simulink model "Simulation_Kinematic_LevMar_InsDiMov"  (R2022a)
settings: Solver=VariableStepAuto  StartTime=0.0  StopTime=0.5  MaxStep=0.01  RelTol=1e-3
values from neighbouring files (symbols this model uses):
  K = 20 * eye(6)    [Kinematic.m]
  mu0 = 1/1000    (= 0.001)    [Kinematic.m]
libraries: robotcorelib x2, robotmaniplib x1
settings Model: Creator=ramti  LastModifiedBy=v
settings SolverCC: AlgebraicLoopSolver=TrustRegion
settings DebuggingCC: UnconnectedInputMsg=warning  UnconnectedOutputMsg=warning  UnconnectedLineMsg=warning  SFMachineParentedDataDiag=warning
settings RTWCC: DLArmComputeVersion=19.05

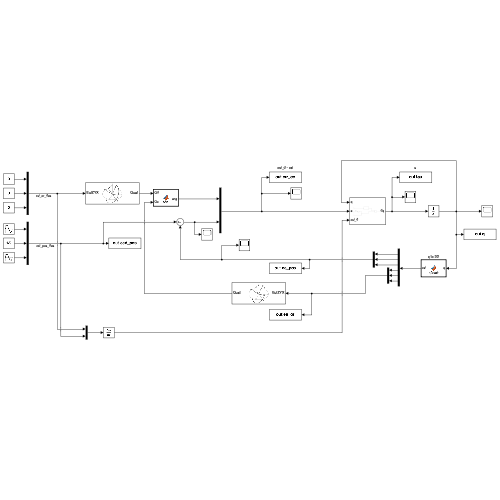
[thumbnail: Simulink's stored preview of the top-level diagram]
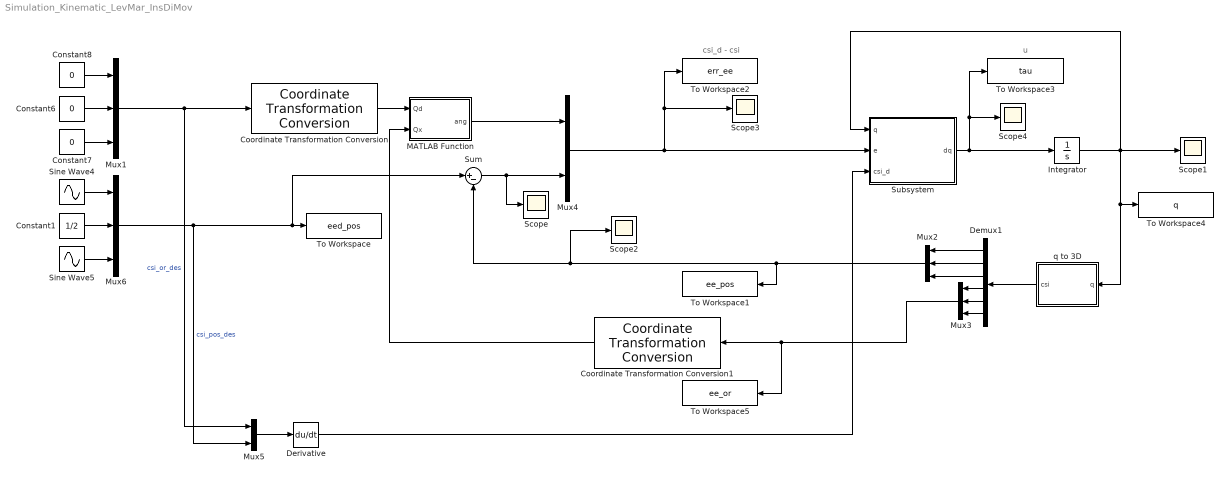
== system Simulation_Kinematic_LevMar_InsDiMov ==
  note: csi_d - csi
  note: u
  Constant1 : Constant  Value=1/2
  Constant6 : Constant  Value=0
  Constant7 : Constant  Value=0
  Constant8 : Constant  Value=0
  Coordinate Transformation Conversion : robotcorelib/Coordinate Transformation Conversion  InputRepresentation=Euler Angles  InputEulerSequence=ZYX  ShowTrVecInputPort=on  OutputRepresentation=Quaternion  OutputEulerSequence=ZYX  ShowTrVecOutputPort=on  SimulateUsing=Interpreted execution
      settings: SourceProductBaseCode=RO,NV,RR,UV
  Coordinate Transformation Conversion1 : robotcorelib/Coordinate Transformation Conversion  InputRepresentation=Euler Angles  InputEulerSequence=ZYX  ShowTrVecInputPort=on  OutputRepresentation=Quaternion  OutputEulerSequence=ZYX  ShowTrVecOutputPort=on  SimulateUsing=Interpreted execution
      settings: SourceProductBaseCode=RO,NV,RR,UV
  Demux1 : Demux  Outputs=6
  Derivative : Derivative
  Integrator : Integrator  InitialCondition=zeros(6,1)
  MATLAB Function : MATLAB Function  TreatAsAtomicUnit=on
  Mux{1..3,6} (4 alike) : Mux  Inputs=3
  Mux4 : Mux  Inputs=2
  Mux5 : Mux  Inputs=2
  Scope{,1..4} (5 alike) : Scope
  Sine Wave4 : Sin  Amplitude=1/2  Frequency=pi/3  SampleTime=0
  Sine Wave5 : Sin  Amplitude=1/2  Frequency=pi/3  Phase=pi/2  SampleTime=0
  Subsystem : Subsystem
      settings: OpenFcn="mdl_puma560_simpl;    % Modello Peter Corke semplificato"
  Sum : Sum  Inputs=|+-
  To Workspace : ToWorkspace  VariableName=eed_pos  SaveFormat=Timeseries  SampleTime=-1
  To Workspace1 : ToWorkspace  VariableName=ee_pos  SaveFormat=Structure With Time  SampleTime=-1
  To Workspace2 : ToWorkspace  VariableName=err_ee  SaveFormat=Structure With Time  SampleTime=-1
  To Workspace3 : ToWorkspace  VariableName=tau  SaveFormat=Structure With Time  SampleTime=-1
  To Workspace4 : ToWorkspace  VariableName=q  SaveFormat=Structure With Time  SampleTime=-1
  To Workspace5 : ToWorkspace  VariableName=ee_or  SaveFormat=Structure With Time  SampleTime=-1
  q to 3D : MATLAB Function  TreatAsAtomicUnit=on
  wires:
  Sum/1 -> Scope/1, Mux4/2
  Demux1/1 -> Mux2/1
  Mux4/1 -> Scope3/1, To Workspace2/1, Subsystem/2(e)
  Demux1/6 -> Mux3/3
  Demux1/5 -> Mux3/2
  MATLAB Function/1(ang) -> Mux4/1
  Demux1/2 -> Mux2/2
  Integrator/1 -> Scope1/1, To Workspace4/1, q to 3D/1(q), Subsystem/1(q)
  Demux1/4 -> Mux3/1
  Demux1/3 -> Mux2/3
  q to 3D/1(csi) -> Demux1/1
  Coordinate Transformation Conversion1/1 -> MATLAB Function/2(Qx)
  Coordinate Transformation Conversion/1 -> MATLAB Function/1(Qd)
  Derivative/1 -> Subsystem/3(csi_d)
  Mux5/1 -> Derivative/1
  Mux6/1 -> Mux5/2, To Workspace/1, Sum/1  "csi_pos_des"
  Subsystem/1(dq) -> Scope4/1, To Workspace3/1, Integrator/1
  Mux2/1 -> To Workspace1/1, Scope2/1, Sum/2
  Mux3/1 -> To Workspace5/1, Coordinate Transformation Conversion1/1
  Sine Wave5/1 -> Mux6/3
  Sine Wave4/1 -> Mux6/1
  Constant1/1 -> Mux6/2
  Constant7/1 -> Mux1/3
  Constant6/1 -> Mux1/2
  Constant8/1 -> Mux1/1
  Mux1/1 -> Mux5/1, Coordinate Transformation Conversion/1  "csi_or_des"

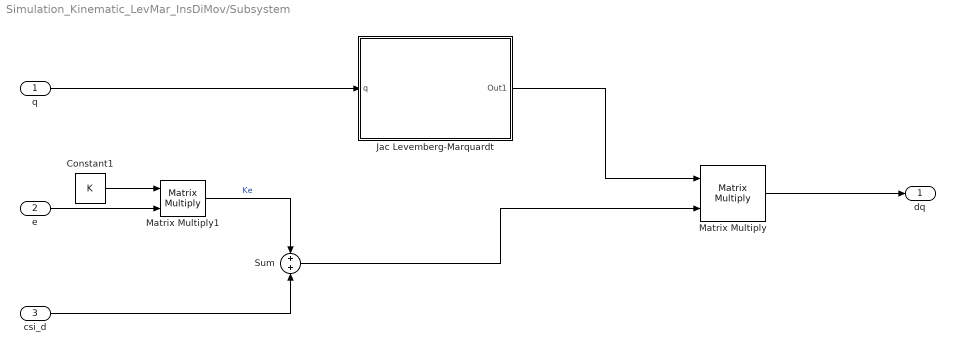
== system Simulation_Kinematic_LevMar_InsDiMov/Subsystem ==
  q : Inport
  e : Inport  Port=2
  csi_d : Inport  Port=3
  Constant1 : Constant  Value=K  VectorParams1D=off
  Jac Levemberg-Marquardt : Subsystem
  Matrix Multiply : Product  Inputs=**  Multiplication=Matrix(*)
  Matrix Multiply1 : Product  Multiplication=Matrix(*)
  Sum : Sum
  dq : Outport
  wires:
  Jac Levemberg-Marquardt/1(Out1) -> Matrix Multiply/1
  Matrix Multiply/1 -> dq/1
  q/1 -> Jac Levemberg-Marquardt/1(q)
  Matrix Multiply1/1 -> Sum/1  "Ke"
  csi_d/1 -> Sum/2
  Sum/1 -> Matrix Multiply/2
  e/1 -> Matrix Multiply1/2
  Constant1/1 -> Matrix Multiply1/1

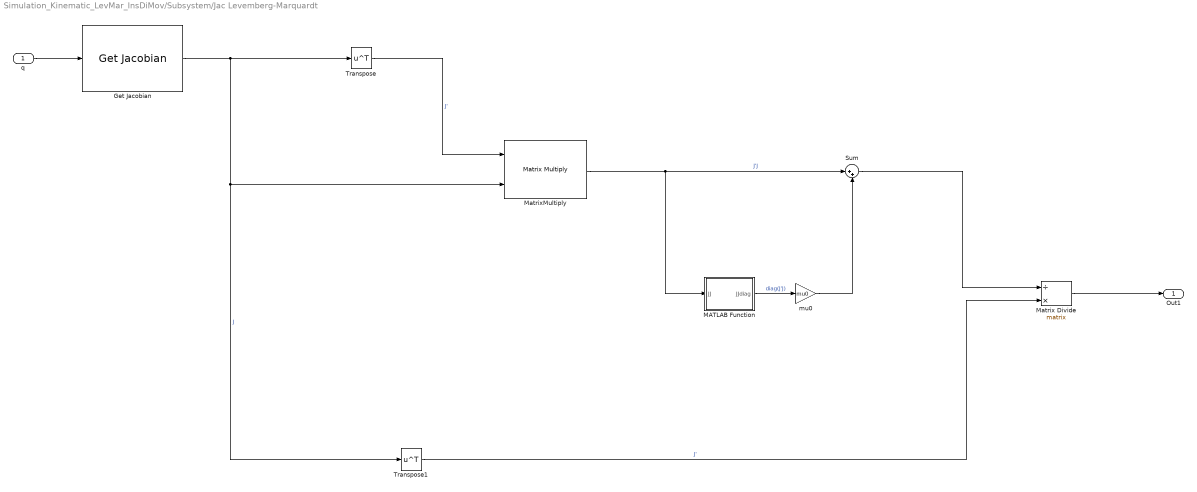
== system Simulation_Kinematic_LevMar_InsDiMov/Subsystem/Jac Levemberg-Marquardt ==
  q : Inport
  Get Jacobian : robotmaniplib/Get Jacobian  RigidBodyTree=robot_p560  EndEffector=body6  SimulateUsing=Interpreted execution
      settings: SourceProductBaseCode=RO
  MATLAB Function : MATLAB Function  TreatAsAtomicUnit=on
  Matrix Divide : Product  Inputs=/*  Multiplication=Matrix(*)
  MatrixMultiply : Product  Multiplication=Matrix(*)
  Sum : Sum  Inputs=|++
  Transpose : Math  Operator=transpose
  Transpose1 : Math  Operator=transpose
  mu0 : Gain  Gain=mu0
  Out1 : Outport
  wires:
  Transpose/1 -> MatrixMultiply/1  "J'"
  MatrixMultiply/1 -> MATLAB Function/1(JJ), Sum/1  "J'J"
  Sum/1 -> Matrix Divide/1
  Get Jacobian/1 -> Transpose1/1, MatrixMultiply/2, Transpose/1  "J"
  Transpose1/1 -> Matrix Divide/2  "J'"
  Matrix Divide/1 -> Out1/1
  MATLAB Function/1(JJdiag) -> mu0/1  "diag(J'J)"
  mu0/1 -> Sum/2
  q/1 -> Get Jacobian/1

== matlab function Simulation_Kinematic_LevMar_InsDiMov/q to 3D ==
  data: q input; csi output
function csi = q2cart(q)

% coder.extrinsic('eval','rotm2eul');

csi = zeros(6,1);

q1 = q(1); q2 = q(2); q3 = q(3); q4 = q(4); q5 = q(5); q6 = q(6); 

% dh = [0 0 0 q1; 0 -pi/2 0 q2; 0.432 0 0.149 q3; 0.0203 -pi/2 0 q4; 0 pi/2 0.433 q5; 0 -pi/2 0 q6];
% Denavit-Hartenberg
a2 = 0.4318;    a3 = 0.0203;
d3 = 0.15005;   d4 = 0.4318;
    
dh = [0     pi/2        0       q1;
      a2    0           0       q2;
      a3    -pi/2       d3      q3;
      0     pi/2        d4      q4;
      0     -pi/2       0       q5;
      0     0           0       q6];
  
A00 = eye(4);

A1 = [cos(dh(1,4)), -sin(dh(1,4))*cos(dh(1,2)), sin(dh( 1,4))*sin(dh( 1,2)),  dh( 1,1)*cos(dh( 1,4)); sin(dh( 1,4)), cos(dh( 1,4))*cos(dh( 1,2)), -cos(dh( 1,4))*sin(dh( 1,2)), dh( 1,1)*sin(dh( 1,4));0, sin(dh( 1,2)), cos(dh( 1,2)), dh(1,3);0, 0, 0, 1];
A2 = [cos(dh(2,4)), -sin(dh(2,4))*cos(dh(2,2)), sin(dh( 2,4))*sin(dh( 2,2)),  dh( 2,1)*cos(dh( 2,4)); sin(dh( 2,4)), cos(dh( 2,4))*cos(dh( 2,2)), -cos(dh( 2,4))*sin(dh( 2,2)), dh( 2,1)*sin(dh( 2,4));0, sin(dh( 2,2)), cos(dh( 2,2)), dh(2,3);0, 0, 0, 1];
A3 = [cos(dh(3,4)), -sin(dh(3,4))*cos(dh(3,2)), sin(dh( 3,4))*sin(dh( 3,2)),  dh( 3,1)*cos(dh( 3,4)); sin(dh( 3,4)), cos(dh( 3,4))*cos(dh( 3,2)), -cos(dh( 3,4))*sin(dh( 3,2)), dh( 3,1)*sin(dh( 3,4));0, sin(dh( 3,2)), cos(dh( 3,2)), dh(3,3);0, 0, 0, 1];
A4 = [cos(dh(4,4)), -sin(dh(4,4))*cos(dh(4,2)), sin(dh( 4,4))*sin(dh( 4,2)),  dh( 4,1)*cos(dh( 4,4)); sin(dh( 4,4)), cos(dh( 4,4))*cos(dh( 4,2)), -cos(dh( 4,4))*sin(dh( 4,2)), dh( 4,1)*sin(dh( 4,4));0, sin(dh( 4,2)), cos(dh( 4,2)), dh(4,3);0, 0, 0, 1];
A5 = [cos(dh(5,4)), -sin(dh(5,4))*cos(dh(5,2)), sin(dh( 5,4))*sin(dh( 5,2)),  dh( 5,1)*cos(dh( 5,4)); sin(dh( 5,4)), cos(dh( 5,4))*cos(dh( 5,2)), -cos(dh( 5,4))*sin(dh( 5,2)), dh( 5,1)*sin(dh( 5,4));0, sin(dh( 5,2)), cos(dh( 5,2)), dh(5,3);0, 0, 0, 1];
A6 = [cos(dh(6,4)), -sin(dh(6,4))*cos(dh(6,2)), sin(dh( 6,4))*sin(dh( 6,2)),  dh( 6,1)*cos(dh( 6,4)); sin(dh( 6,4)), cos(dh( 6,4))*cos(dh( 6,2)), -cos(dh( 6,4))*sin(dh( 6,2)), dh( 6,1)*sin(dh( 6,4));0, sin(dh( 6,2)), cos(dh( 6,2)), dh(6,3);0, 0, 0, 1];

A06 = A00*A1*A2*A3*A4*A5*A6;

% for (i=1:6)
%    
%     eval(sprintf('A%d= [cos(dh(%d,4)), -sin(dh(%d,4))*cos(dh(%d,2)), sin(dh( %d,4))*sin(dh( %d,2)),  dh( %d,1)*cos(dh( %d,4)); sin(dh( %d,4)), cos(dh( %d,4))*cos(dh( %d,2)), -cos(dh( %d,4))*sin(dh( %d,2)), dh( %d,1)*sin(dh( %d,4));0, sin(dh( %d,2)), cos(dh( %d,2)), dh(%d,3);0, 0, 0, 1];',i*ones(1,18)))
% 
%     eval(sprintf('A0%d = A0%d*A%d;',i,i-1,i))
% end

xi_hom = A06*[0;0;0;1];

R_xi = A06(1:3,1:3);
csi = [xi_hom(1:3);transpose(rotm2eul(R_xi))];

== matlab function Simulation_Kinematic_LevMar_InsDiMov/MATLAB Function ==
  data: Qd input; ang output; Qx input
function ang = fcn(Qd, Qx)

%% 1 
% Qx_cj = [Qx(1);-Qx(2:4)];
% 
% Qr = [Qd(1)*Qx_cj(1)-dot(Qd(2:4),Qx_cj(2:4));Qd(1)*Qx_cj(2:4)+Qx_cj(1)*Qd(2:4)+cross(Qd(2:4),Qx_cj(2:4))];
% 
% if (Qr(1)==0)
%     ang=[Qr(4);Qr(3);Qr(2)];
% else
%     ang = sign(Qr(1))*[Qr(4);Qr(3);Qr(2)];
% end

%% 2
% ang = Qd(1)*Qx(2:4) - Qx(1)*Qd(2:4) - cross(Qd(2:4),Qx(2:4));

%% 3
Rd = quat2rotm(transpose(Qd));
Rx = quat2rotm(transpose(Qx));

% Re = Rd*transpose(Rx);

% e = rotm2quat(Re);
% 
% ang = transpose(2*e(1)*e(2:4));

ang = (cross(Rd(:,1),Rx(:,1)) + cross(Rd(:,2),Rx(:,2)) +cross(Rd(:,3),Rx(:,3)))/2;

%% 4
% Rd = quat2rotm(transpose(Qd));
% Rx = quat2rotm(transpose(Qx));
% 
% Re = transpose(Rx)*Rd;
% 
% qer = rotm2quat(Re);
% ang = Rx*transpose(qer(2:4));

== matlab function Simulation_Kinematic_LevMar_InsDiMov/Subsystem/Jac Levemberg-Marquardt/MATLAB Function ==
  data: JJ input; JJdiag output
function JJdiag = diagonale(JJ)

v = diag(JJ);

JJdiag = diag(v);
